simulink model "dyn"  (R2025b)
settings: Solver=FixedStepDiscrete  StartTime=0.0  StopTime=inf  FixedStep=128/48000  RelTol=1e-3
model workspace (MATLAB code in the model file):
  | Gain_rt = Simulink.Parameter(1.0);
  | Bypass_rt = Simulink.Parameter(false);
undefined symbols (not defined in the file): Attack_rt, Knee_rt, Makeup_rt, Mix_rt, Ratio_rt, Release_rt, Threshold_rt
settings Model: Creator=linogarciamorales  LastModifiedBy=linogarciamorales
settings OptimizationCC: EnhancedBackFolding=on  PassReuseOutputArgsAs=Individual arguments  ZeroExternalMemoryAtStartup=off  ZeroInternalMemoryAtStartup=off  OptimizeBlockOrder=speed  DifferentSizesBufferReuse=on  OptimizationCustomize=off  EfficientTunableParamExpr=on
settings DebuggingCC: ParameterTunabilityLossMsg=error
settings SFSimCC: MATLABDynamicMemAlloc=off
settings RTWCC: SystemTargetFile=ert.tlc  GenCodeOnly=on  TemplateMakefile=ert_default_tmf  Description=Embedded Coder
settings CodeAppCC: ForceParamTrailComments=on  IgnoreCustomStorageClasses=off  OperatorAnnotations=on  SimulinkDataObjDesc=on  SFDataObjDesc=on  InsertBlockDesc=on
settings ERTTargetCC: InlinedParameterPlacement=Hierarchical  ERTCustomFileTemplate=example_file_process.tlc  TargetLangStandard=C99 (ISO)  GenerateSampleERTMain=on  SupportNonInlinedSFcns=on

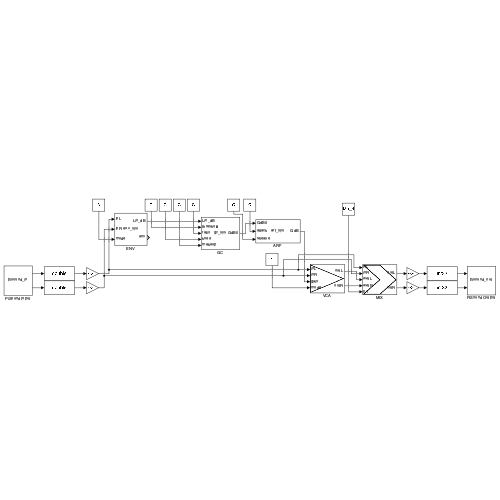
[thumbnail: Simulink's stored preview of the top-level diagram]
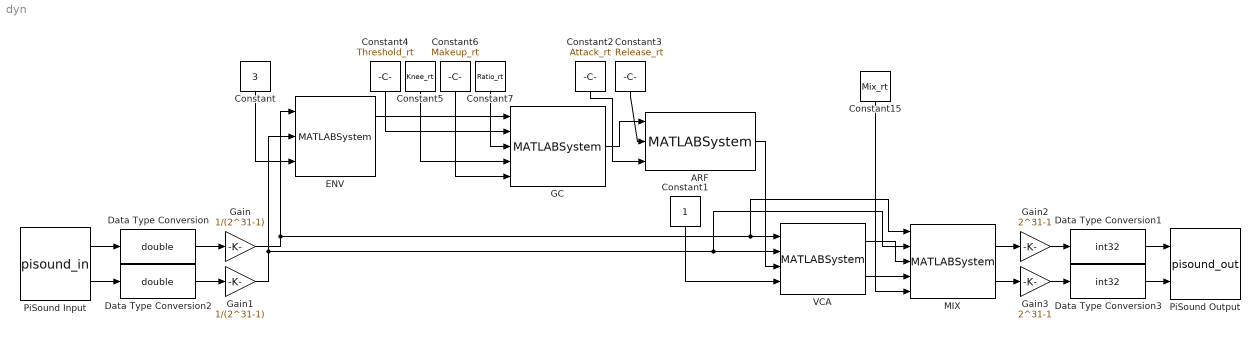
== system dyn ==
  ARF : MATLABSystem  System=arf_sys  N=128  Fs=48000  AttackDefault=0.010  ReleaseDefault=0.100  SimulateUsing=Code generation
      mask Type: arf_sys
  Constant : Constant  Value=3  OutDataTypeStr=uint8
  Constant1 : Constant  OutDataTypeStr=uint8
  Constant15 : Constant  Value=Mix_rt  OutDataTypeStr=double
  Constant2 : Constant  Value=Attack_rt  OutDataTypeStr=double
  Constant3 : Constant  Value=Release_rt  OutDataTypeStr=double
  Constant4 : Constant  Value=Threshold_rt  OutDataTypeStr=double
  Constant5 : Constant  Value=Knee_rt  OutDataTypeStr=double
  Constant6 : Constant  Value=Makeup_rt  OutDataTypeStr=double
  Constant7 : Constant  Value=Ratio_rt  OutDataTypeStr=double
  Data Type Conversion : DataTypeConversion  OutDataTypeStr=double  SaturateOnIntegerOverflow=off  RndMeth=Floor
  Data Type Conversion1 : DataTypeConversion  OutDataTypeStr=int32  SaturateOnIntegerOverflow=off  RndMeth=Floor
  Data Type Conversion2 : DataTypeConversion  OutDataTypeStr=double  SaturateOnIntegerOverflow=off  RndMeth=Floor
  Data Type Conversion3 : DataTypeConversion  OutDataTypeStr=int32  SaturateOnIntegerOverflow=off  RndMeth=Floor
  ENV : MATLABSystem  System=env_sys  N=128  Fs=48000  ModeDefault=uint8( 1 )  Eps=1e-12  TauRMS=0.02  SimulateUsing=Code generation
      mask Type: env_sys
  GC : MATLABSystem  System=gc_sys  N=128  Eps=1e-12  Floor_dB=-80  SimulateUsing=Code generation
      mask Type: gc_sys
  Gain : Gain  Gain=1/(2^31-1)
  Gain1 : Gain  Gain=1/(2^31-1)
  Gain2 : Gain  Gain=2^31-1
  Gain3 : Gain  Gain=2^31-1
  MIX : MATLABSystem  System=mix_sys  N=128  Fs=48000  Mode=uint8( 0 )  SmoothTime=0.01  IndepInDB=false  SimulateUsing=Code generation
      mask Type: mix_sys
  PiSound Input : S-Function  FunctionName=pisound_in  Parameters=48000, 128, 0  SFunctionDeploymentMode=off  EnableBusSupport=off
  PiSound Output : S-Function  FunctionName=pisound_out  Parameters=48000, 128, 0  SFunctionDeploymentMode=off  EnableBusSupport=off
  VCA : MATLABSystem  System=vca_sys  N=128  Fs=48000  bypass=uint8(0)  SimulateUsing=Code generation
      mask Type: vca_sys
  wires:
  PiSound Input/1 -> Data Type Conversion/1
  PiSound Input/2 -> Data Type Conversion2/1
  Data Type Conversion1/1 -> PiSound Output/1
  Data Type Conversion3/1 -> PiSound Output/2
  Gain2/1 -> Data Type Conversion1/1
  Gain3/1 -> Data Type Conversion3/1
  Data Type Conversion/1 -> Gain/1
  Data Type Conversion2/1 -> Gain1/1
  Gain/1 -> ENV/1, MIX/1, VCA/1
  Gain1/1 -> MIX/2, VCA/2, ENV/2
  Constant/1 -> ENV/3
  ENV/1 -> GC/1
  ARF/1 -> VCA/3
  Constant1/1 -> VCA/4
  GC/1 -> ARF/1
  Constant2/1 -> ARF/3
  Constant3/1 -> ARF/2
  Constant5/1 -> GC/4
  Constant4/1 -> GC/2
  Constant6/1 -> GC/5
  Constant7/1 -> GC/3
  VCA/1 -> MIX/3
  VCA/2 -> MIX/4
  MIX/1 -> Gain2/1
  MIX/2 -> Gain3/1
  Constant15/1 -> MIX/5
